simulink model "PI_TeC_PIControl"  (R2020a)
settings: Solver=FixedStepAuto  StartTime=0.0  StopTime=inf  RelTol=1e-3  EnableMultiTasking=on
libraries: arduinolib x2, simulink x1
Description:
  | Temperature control model using ON/OFF control.
settings Model: SILPILModeSetting=veronly  ExtModeTrigDuration=2  Creator=Mohanad M. Marzouk  LastModifiedBy=Mohanad M. Marzouk
settings SolverCC: PositivePriorityOrder=on
settings OptimizationCC: EnhancedBackFolding=on  PassReuseOutputArgsAs=Individual arguments  ZeroExternalMemoryAtStartup=off  ZeroInternalMemoryAtStartup=off  MaxStackSize=64  OptimizeBlockOrder=speed  DifferentSizesBufferReuse=on  OptimizationCustomize=off  EfficientTunableParamExpr=on
settings DebuggingCC: ParameterTunabilityLossMsg=error  SFMachineParentedDataDiag=error
settings HardwareCC: ProdBitPerInt=16  ProdBitPerPointer=16  ProdBitPerSizeT=16  ProdBitPerPtrDiffT=16  ProdLargestAtomicFloat=None  ProdWordSize=8  ProdHWDeviceType=Atmel->AVR
settings RTWCC: SystemTargetFile=ert.tlc  HardwareBoard=Arduino Uno  TLCOptions="-aInlineSetEventsForThisBaseRateFcn=TLC_FALSE -aSuppressMultiTaskScheduler=TLC_FALSE   -aRateBasedStepFcn=1"  TemplateMakefile=ert_default_tmf  GenerateReport=on  Toolchain=Arduino AVR  BuildConfiguration=Faster Runs
settings CodeAppCC: ForceParamTrailComments=on  IgnoreCustomStorageClasses=off  OperatorAnnotations=on  SimulinkDataObjDesc=on  SFDataObjDesc=on  InsertBlockDesc=on
settings ERTTargetCC: SupportContinuousTime=on  SupportVariableSizeSignals=on  ExtModeStaticAllocSize=250

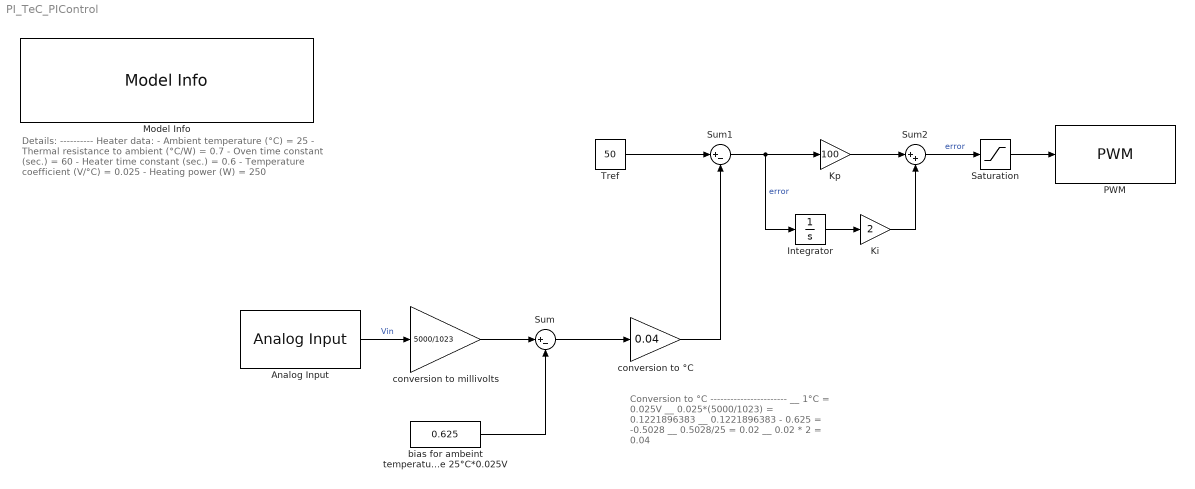
== system PI_TeC_PIControl ==
  note: Details:
      | ----------
      | Heater data:
      | - Ambient temperature (°C) = 25
      | - Thermal resistance to ambient (°C/W) = 0.7
      | - Oven time constant (sec.) = 60
      | - Heater time constant (sec.) = 0.6
      | - Temperature coefficient (V/°C) = 0.025
      | - Heating power (W) = 250
  note: Conversion to °C
      | -----------------------
      | __ 1°C = 0.025V
      | __ 0.025*(5000/1023) = 0.1221896383
      | __ 0.1221896383 - 0.625 = -0.5028
      | __ 0.5028/25 = 0.02
      | __ 0.02 * 2 = 0.04
  Analog Input : arduinolib/Analog Input  pinNumber=0  ReadResultsOnly=off  ConversionTriggerSource=Software  ExternalTriggerType=uint32( 0 )  OutputDataType=uint16  EnableConversionCompleteNotify=off  EnableOuputStatus=off  SampleTime=-1  blockPlatform=arduino
  Integrator : Integrator
  Ki : Gain  Gain=2
  Kp : Gain  Gain=100
  Model Info : simulink/Model-Wide Utilities/Model Info  Frame=on  DisplayStringWithTags=|  HorizontalTextAlignment=Left  LeftAlignmentValue=0.02
      | Model Info
      | ------------------------------------------------------------------------------
      | @model	:		%<ModelName>
      | @version	:		%<ModelVersion>
      | @author	:		%<Creator>
      | @brief	:		%<Description>
  PWM : arduinolib/PWM  pinNumber=9  frequencyType=Default  desiredFrequency=490.2  achievableFrequency=490.2
  Saturation : Saturate  UpperLimit=255  LowerLimit=0
  Sum : Sum  Inputs=|+-
  Sum1 : Sum  Inputs=|+-
  Sum2 : Sum  Inputs=|++
  Tref : Constant  Value=50
  bias for ambeint temperature 25°C*0.025V : Constant  Value=0.625
  conversion to millivolts : Gain  Gain=5000/1023
  conversion to °C : Gain  Gain=0.04
  wires:
  Analog Input/1 -> conversion to millivolts/1  "Vin"
  conversion to °C/1 -> Sum1/2
  Tref/1 -> Sum1/1
  Saturation/1 -> PWM/1
  conversion to millivolts/1 -> Sum/1
  Sum/1 -> conversion to °C/1
  bias for ambeint temperature 25°C*0.025V/1 -> Sum/2
  Sum1/1 -> Integrator/1, Kp/1  "error"
  Integrator/1 -> Ki/1
  Kp/1 -> Sum2/1
  Ki/1 -> Sum2/2
  Sum2/1 -> Saturation/1  "error"
